simulink model "Copy_of_MPC_control"  (R2018a)
settings: Solver=FixedStepAuto  StartTime=0  StopTime=Tend  FixedStep=0.001  RelTol=5e-3
model workspace (MAT data in the model file):
  A_mu = 10
  B_reff = 8.386
  Cz = 7766.25
  DCT_Param : struct (value not decoded)
  D_reff = 0.25826
  Downshift_Speeds = [9.5625 12.9375 16.3125 19.6875 23.0625 26.4375 29.8125 33.1875 36.5625 39.9375 43.3125 46.6875 ... (28 elements, 4x7)]
  Pedal_Positions = [0.1 0.4 0.5 0.9]
  SUS : struct (value not decoded)
  Upshift_Speeds = [12.9375 16.3125 19.6875 33 26.4375 29.8125 33.1875 52.5 39.9375 43.3125 46.6875 77.25 ... (28 elements, 4x7)]
  VEH : struct (value not decoded)
  V_o = 16.7
  V_xlow = 1
  WH : struct (value not decoded)
  a = 1.4
  alpha_max = 1.5
  alpha_min = -1.5
  b = 1.8
  c_zo = 209651
  epsilon = 0.1
  h = 0.134
  path : struct (value not decoded)
  pio = 220000
  q_Fcx = 0
  q_Fz2 = 15.4
  q_Fzy = 0
  q_reo = 0.9974
  q_sx1 = -0.007764
  q_sx10 = 0.2824
  q_sx11 = 5.349
  q_sx12 = 0
  q_sx13 = 0
  q_sx14 = 0
  q_sx2 = 1.1915
  q_sx3 = 0.013948
  q_sx4 = 4.912
  q_sx5 = 1.02
  q_sx6 = 22.83
  q_sx7 = 0.7104
  q_sx8 = -0.023393
  q_sx9 = 0.6581
  q_sy1 = 0.00702
  q_sy2 = 0
  q_sy3 = 0.001515
  q_sy4 = 8.514e-05
  q_sy5 = 0
  q_sy6 = 0
  q_sy7 = 0.9008
  q_sy8 = -0.4089
  q_v1 = 0.0007742
  q_v2 = 0.04667
  r_Bx1 = 12.531
  r_Bx2 = 9.532
  r_Bx3 = 0
  r_By1 = 10.615
  r_By2 = 7.705
  r_By3 = 3.433e-06
  r_By4 = 0
  r_Cx1 = 1.019
  r_Cy1 = 1.0585
  r_Ex1 = -0.4487
  r_Ex2 = -0.4726
  r_Ey1 = 0.3132
  r_Ey2 = 7.63e-06
  r_Hx1 = 0.0002374
  r_Hy1 = 0.011646
  r_Hy2 = 7.63e-06
  r_Vy1 = 0.05654
  r_Vy2 = 7.63e-06
  r_Vy3 = 0
  r_Vy4 = 99.9
  r_Vy5 = 2
  r_Vy6 = 15.814
  r_o = 0.3135
  vehWidth = 2
  w = 1
symbols that are objects in the model workspace (value not decoded): VEH
undefined symbols (not defined in the file): C_Brake, C_Final, C_Front, C_Front_1, C_Front_2, C_Middle, C_out_Brake, C_out_Final, C_out_Front, C_out_Front_1, C_out_Front_2, C_out_Middle, Co, Cok_Brake, Cok_Final, Cok_Front_1, Cok_Front_2, Cok_Middle, Cso, D_out_Brake, D_out_Final, D_out_Front, D_out_Front_1, D_out_Front_2, D_out_Middle, Earlytochange, Earlytochange2, F, F_Brake, F_Final, F_Front, F_Front_1, F_Front_2, F_Middle, Fs, G_Brake, G_Final, G_Front_1, G_Front_2, G_Middle, G_sys_Brake, G_sys_Final, G_sys_Front, G_sys_Front_1, G_sys_Front_2, G_sys_Middle, Gd, Gd_Brake, Gd_Final, Gd_Front, Gd_Front_1, Gd_Front_2, Gd_Middle, Go, Gsd, Gso, H_Brake, H_Final, H_Front_1, H_Front_2 ... (+60)
libraries: simulink x10, sim3dlib x4, autolibutils x2, vehdynlibviscommon x2
(part 4 of 8)

== system Copy_of_MPC_control/Visualization/3D Engine/3D Engine ==
  VehFdbk : Inport
  3D Body Offset : Constant  Value=single(0.0112)  OutDataTypeStr=single
  Add1 : Sum  Inputs=-+
  Add3 : Sum  Inputs=-+-
  Bus Selector : BusSelector  OutputSignals=Body.X,Body.Y,Body.Z,Body.phi,Body.theta,Body.psi
  Bus Selector2 : BusSelector  OutputSignals=Wheels.zAxle,Wheels.omega,Driveline.WhlAng
  Bus Selector3 : BusSelector  OutputSignals=Body.ZHP
  Constant1 : Constant  Value=zeros(4,1)  OutDataTypeStr=single
  Constant2 : Constant  Value=0  OutDataTypeStr=single
  Constant8 : Constant  Value=h
  Data Type Conversion{1,4..10,12} (9 alike) : DataTypeConversion  OutDataTypeStr=single
  Demux{,1..3} (4 alike) : Demux
  Integrator : Integrator  WrapState=on  WrappedStateUpperValue=2*pi  WrappedStateLowerValue=0  ZeroCross=off
  Part Rotation Concatenation : Subsystem
  Part Translation Concatenation : Subsystem
  Rate Transition : RateTransition  OutPortSampleTime=dt3D
  Scale : Subsystem
  Simulation 3D Engine 1 : sim3dlib/Simulation 3D Config  Priority=1  ProjectFormat=Executable  ProjectName=VehicleSimulation.exe  SceneDesc=Straight road  OpVisEn=off  Ts=dt3D
      settings: AttributesFormatString=Priority: %<Priority>
  Unary Minus : UnaryMinus
  Vehicle Actor Transform Set : sim3dlib/Simulation 3D Actor Transform Set  ActorTag=SimulinkVehicle1  ActorType=Passenger vehicle  PassVehMesh=Muscle car  VehColor=Red  NumberOfParts=5  CustNumOfParts=3  Translation=[0 0 1; 0 0 0; 0 0 0; 0 0 0; 0 0 0]  Rotation=[0 0 0; 0 0 0; 0 0 0; 0 0 0; 0 0 0]  Scale=[1 1 1; 1 1 1; 1 1 1; 1 1 1; 1 1 1]  Ts=dt3D
  wires:
  Unary Minus/1 -> Integrator/1
  Bus Selector3/1 -> Add3/2  "<ZHP>"
  Add3/1 -> Data Type Conversion12/1
  Bus Selector2/1 -> Add3/3  "<zAxle>"
  Constant8/1 -> Add3/1
  Rate Transition/1 -> Bus Selector/1, Bus Selector3/1, Bus Selector2/1
  Scale/1(ScaleOut) -> Vehicle Actor Transform Set/3
  Demux/4 -> Part Rotation Concatenation/7(WheelRearRight Ptich)
  Demux/3 -> Part Rotation Concatenation/6(WheelRearLeft Pitch)
  Demux/2 -> Part Rotation Concatenation/5(WheelFrontRight Pitch)
  Demux/1 -> Part Rotation Concatenation/4(WheelFrontLeft Pitch)
  Constant1/1 -> Demux2/1
  Bus Selector/4 -> Data Type Conversion7/1  "<phi>"
  Data Type Conversion6/1 -> Add1/1
  Part Rotation Concatenation/1(ConcatOut) -> Vehicle Actor Transform Set/2
  Part Translation Concatenation/1(ConcatOut) -> Vehicle Actor Transform Set/1
  Data Type Conversion12/1 -> Demux3/1
  Demux3/4 -> Part Translation Concatenation/15(WheelRearRightZ)
  Demux3/3 -> Part Translation Concatenation/14(WheelRearLeftZ)
  Demux3/1 -> Part Translation Concatenation/12(WheelFrontLeftZ)
  Demux3/2 -> Part Translation Concatenation/13(WheelFrontRightZ)
  VehFdbk/1 -> Rate Transition/1
  Add1/1 -> Part Translation Concatenation/3(BodyZ)
  3D Body Offset/1 -> Add1/2
  Demux1/4 -> Part Rotation Concatenation/15(WheelRearRight Yaw)
  Demux1/3 -> Part Rotation Concatenation/14(WheelRearLeft Yaw)
  Demux2/1 -> Part Rotation Concatenation/8(WheelFrontLeft Roll)
  Demux2/2 -> Part Rotation Concatenation/9(WheelFrontRight Roll)
  Demux2/3 -> Part Rotation Concatenation/10(WheelRearLeft Roll)
  Demux2/4 -> Part Rotation Concatenation/11(WheelRearRight Roll)
  Bus Selector2/3 -> Data Type Conversion9/1  "<WhlAng>"
  Bus Selector2/2 -> Unary Minus/1  "<omega>"
  Data Type Conversion9/1 -> Demux1/1
  Demux1/1 -> Part Rotation Concatenation/12(WheelFrontLeft Yaw)
  Demux1/2 -> Part Rotation Concatenation/13(WheelFrontRight Yaw)
  Integrator/1 -> Data Type Conversion1/1
  Data Type Conversion1/1 -> Demux/1
  Data Type Conversion8/1 -> Part Rotation Concatenation/2(Body Ptich)
  Data Type Conversion5/1 -> Part Translation Concatenation/2(BodyY)
  Data Type Conversion10/1 -> Part Rotation Concatenation/3(Body Yaw)
  Constant2/1 -> Part Translation Concatenation/5(WheelFrontRightX), Part Translation Concatenation/6(WheelRearLeftX), Part Translation Concatenation/7(WheelRearRightX), Part Translation Concatenation/8(WheelFrontLeftY), Part Translation Concatenation/9(WheelFrontRightY), Part Translation Concatenation/10(WheelRearLeftY), Part Translation Concatenation/11(WheelRearRightY), Part Translation Concatenation/4(WheelFrontLeftX)
  Data Type Conversion4/1 -> Part Translation Concatenation/1(BodyX)
  Data Type Conversion7/1 -> Part Rotation Concatenation/1(Body Roll)
  Bus Selector/1 -> Data Type Conversion4/1  "<X>"
  Bus Selector/2 -> Data Type Conversion5/1  "<Y>"
  Bus Selector/3 -> Data Type Conversion6/1  "<Z>"
  Bus Selector/6 -> Data Type Conversion10/1  "<psi>"
  Bus Selector/5 -> Data Type Conversion8/1  "<theta>"

== system Copy_of_MPC_control/Visualization/3D Engine/3D Engine Disabled ==
  VehFdbk : Inport
  Terminator : Terminator
  wires:
  VehFdbk/1 -> Terminator/1

== system Copy_of_MPC_control/all_system/Controllers1/Brake Controller ==
  BrkPrsCmd : Inport
  xdot : Inport  Port=2
  kappa : Inport  Port=3
  Abs : Abs  ZeroCross=off
  Brake Pressure Control : Subsystem  Variant=on  OverrideUsingVariant=0
  Constant1 : Constant  Value=-20
  Gain3 : Gain
  Integrator2 : Integrator  LimitOutput=on  UpperSaturationLimit=1  LowerSaturationLimit=0
  Saturation : Saturate  UpperLimit=1  LowerLimit=0  ZeroCross=off
  Switch1 : Switch  Criteria=u2 > Threshold  Threshold=.1
  Vector Concatenate2 : Concatenate  NumInputs=4
  PCmd : Outport
  wires:
  Constant1/1 -> Switch1/3
  Gain3/1 -> Switch1/1
  Saturation/1 -> Brake Pressure Control/3(<Kappa>)  "Kappa"
  Brake Pressure Control/1(PCmd) -> PCmd/1
  kappa/1 -> Abs/1
  Integrator2/1 -> Vector Concatenate2/4, Vector Concatenate2/3, Vector Concatenate2/2, Vector Concatenate2/1
  xdot/1 -> Brake Pressure Control/2(xdot)
  Abs/1 -> Saturation/1
  Vector Concatenate2/1 -> Brake Pressure Control/1(Pref)  "Reference P"
  BrkPrsCmd/1 -> Switch1/2, Gain3/1
  Switch1/1 -> Integrator2/1

== system Copy_of_MPC_control/all_system/Controllers1/ECU ==
  <Accel> : Inport
  Acc to Torque Request : Gain  Gain=150
  Trq Cmd : Outport
  wires:
  <Accel>/1 -> Acc to Torque Request/1
  Acc to Torque Request/1 -> Trq Cmd/1

== system Copy_of_MPC_control/all_system/Controllers1/Transmission Controller ==
  Acc : Inport
  EngSpd : Inport  Port=2  Unit=rad/s
  PropShaftSpd : Inport  Port=3
  10ms Function-Call Generator : simulink/Ports & Subsystems/Function-Call Generator  sample_time=Fcncal_transctrl_Ts  numberOfIterations=1
  Rate Transition{,1..3} (4 alike) : RateTransition
  Signal Specification : SignalSpecification  Unit=rpm
  TCM : Subsystem
  Unit Conversion : UnitConversion
  Gear : Outport
  wires:
  TCM/1(Gear Select) -> Rate Transition3/1
  Rate Transition/1 -> TCM/1(AccCmd)
  10ms Function-Call Generator/1 -> TCM/Trigger
  Acc/1 -> Rate Transition/1
  PropShaftSpd/1 -> Rate Transition2/1
  Rate Transition1/1 -> TCM/2(EngSpd)
  Rate Transition2/1 -> TCM/3(VehSpdFdbk)
  Rate Transition3/1 -> Gear/1
  Unit Conversion/1 -> Signal Specification/1
  Signal Specification/1 -> Rate Transition1/1  "EngSpd"
  EngSpd/1 -> Unit Conversion/1

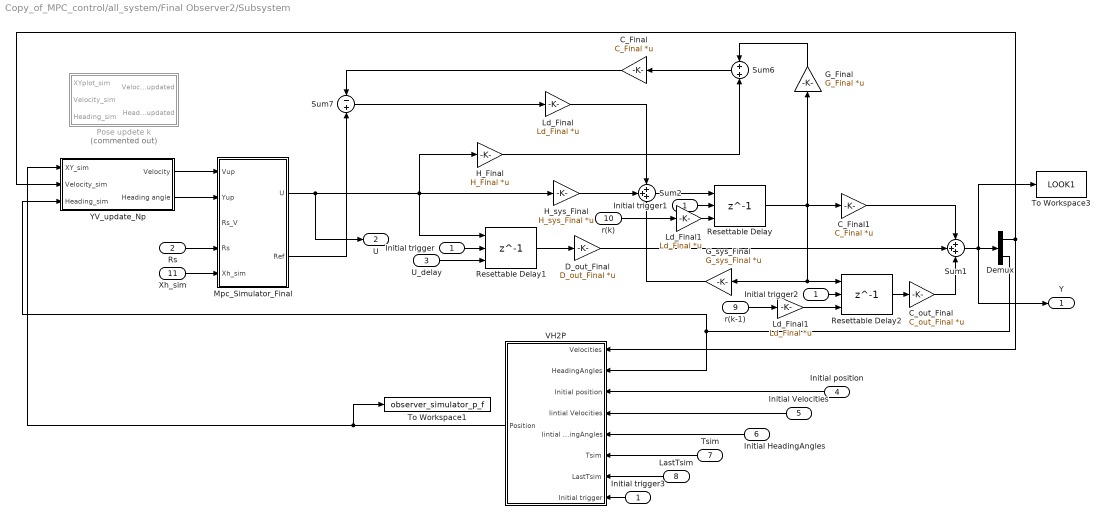
== system Copy_of_MPC_control/all_system/Final Observer2/Subsystem ==
  Initial trigger : Inport
  Rs : Inport  Port=2
  U_delay : Inport  Port=3
  Initial position : Inport  Port=4
  Initial Velocities : Inport  Port=5
  Initial HeadingAngles : Inport  Port=6
  Tsim : Inport  Port=7
  LastTsim : Inport  Port=8
  r(k-1) : Inport  Port=9
  r(k) : Inport  Port=10
  Xh_sim : Inport  Port=11
  C_Final : Gain  Gain=C_Final  Multiplication=Matrix(K*u) (u vector)
  C_Final1 : Gain  Gain=C_Final  Multiplication=Matrix(K*u) (u vector)
  C_out_Final : Gain  Gain=C_out_Final  Multiplication=Matrix(K*u) (u vector)
  D_out_Final : Gain  Gain=D_out_Final  Multiplication=Matrix(K*u) (u vector)
  Demux : Demux  Outputs=2
  G_Final : Gain  Gain=G_Final  Multiplication=Matrix(K*u) (u vector)
  G_sys_Final : Gain  Gain=G_sys_Final  Multiplication=Matrix(K*u) (u vector)
  H_Final : Gain  Gain=H_Final  Multiplication=Matrix(K*u) (u vector)
  H_sys_Final : Gain  Gain=H_sys_Final  Multiplication=Matrix(K*u) (u vector)
  Initial trigger1 : InportShadow
  Initial trigger2 : InportShadow
  Initial trigger3 : InportShadow
  Ld_Final : Gain  Gain=Ld_Final  Multiplication=Matrix(K*u) (u vector)
  Ld_Final1 : Gain  Gain=Ld_Final  Multiplication=Matrix(K*u) (u vector)
  "Ld_Final1 " : Gain  Gain=Ld_Final  Multiplication=Matrix(K*u) (u vector)
  Mpc_Simulator_Final : Subsystem
  Pose updete k : Subsystem  Commented=on
  Resettable Delay : Delay  DelayLength=1  InitialConditionSource=Input port  ExternalReset=Falling  SampleTime=Ts
      settings: InputPortMap=u0,r5,p4
  Resettable Delay1 : Delay  DelayLength=1  InitialConditionSource=Input port  ExternalReset=Falling  SampleTime=Ts
      settings: InputPortMap=u0,r5,p4
  Resettable Delay2 : Delay  DelayLength=1  InitialConditionSource=Input port  ExternalReset=Falling  SampleTime=Ts
      settings: InputPortMap=u0,r5,p4
  Sum1 : Sum  Inputs=+++
  Sum2 : Sum  Inputs=+++
  Sum6 : Sum
  Sum7 : Sum  Inputs=-+
  To Workspace1 : ToWorkspace  VariableName=observer_simulator_p_f  SampleTime=Ts
  To Workspace3 : ToWorkspace  VariableName=LOOK1  SampleTime=Ts
  VH2P : Subsystem
  YV_update_Np : Subsystem  TreatAsAtomicUnit=on
  Y : Outport
  U : Outport  Port=2
  wires:
  U_delay/1 -> Resettable Delay1/3
  Initial position/1 -> VH2P/3(Initial position)
  Mpc_Simulator_Final/1(U) -> U/1, Resettable Delay1/1, H_sys_Final/1, H_Final/1
  Resettable Delay/1 -> G_sys_Final/1, Resettable Delay2/1, C_Final1/1, G_Final/1
  Sum7/1 -> Ld_Final/1
  C_Final1/1 -> Sum1/1
  Rs/1 -> Mpc_Simulator_Final/4(Rs)
  Demux/1 -> YV_update_Np/2(Velocity_sim), VH2P/1(Velocities)
  Demux/2 -> YV_update_Np/3(Heading_sim), VH2P/2(HeadingAngles)
  Resettable Delay1/1 -> D_out_Final/1
  LastTsim/1 -> VH2P/7(LastTsim)
  Ld_Final/1 -> Sum2/1
  Initial Velocities/1 -> VH2P/4(Iintial Velocities)
  D_out_Final/1 -> Sum1/2
  YV_update_Np/1(Velocity) -> Mpc_Simulator_Final/1(Vup)
  r(k)/1 -> "Ld_Final1 "/1
  Resettable Delay2/1 -> C_out_Final/1
  G_sys_Final/1 -> Sum2/3
  r(k-1)/1 -> Ld_Final1/1
  C_Final/1 -> Sum7/1
  Sum2/1 -> Resettable Delay/1
  VH2P/1(Position) -> YV_update_Np/1(XY_sim), To Workspace1/1
  YV_update_Np/2(Heading angle) -> Mpc_Simulator_Final/2(Yup)
  Xh_sim/1 -> Mpc_Simulator_Final/5(Xh_sim)
  Tsim/1 -> VH2P/6(Tsim)
  "Ld_Final1 "/1 -> Resettable Delay/3
  Initial HeadingAngles/1 -> VH2P/5(Iintial HeadingAngles)
  G_Final/1 -> Sum6/1
  H_Final/1 -> Sum6/2
  C_out_Final/1 -> Sum1/3
  Sum1/1 -> Y/1, To Workspace3/1, Demux/1
  Sum6/1 -> C_Final/1
  Mpc_Simulator_Final/2(Ref) -> Sum7/2
  H_sys_Final/1 -> Sum2/2
  Ld_Final1/1 -> Resettable Delay2/3
  Initial trigger/1 -> Resettable Delay1/2
  Initial trigger1/1 -> Resettable Delay/2
  Initial trigger2/1 -> Resettable Delay2/2
  Initial trigger3/1 -> VH2P/8(Initial trigger)

== system Copy_of_MPC_control/all_system/Final_simulator1/Mpc_Simulator_Final ==
  Vup : Inport  SampleTime=Ts  LockScale=on
  Yup : Inport  Port=2  SampleTime=Ts  LockScale=on
  Rs_V : Inport  Port=3  SampleTime=Ts  LockScale=on
  Rs : Inport  Port=4  SampleTime=Ts  LockScale=on
  Xh_sim : Inport  Port=5
  Clock : Clock
  Constant1 : Constant  Value=M  VectorParams1D=off  SampleTime=-1
  Constant2 : Constant  Value=Np  SampleTime=-1
  Constant3 : Constant  Value=Upd_end  VectorParams1D=off  SampleTime=-1
  Constant4 : Constant  Value=Qc  VectorParams1D=off  SampleTime=-1
  Constant5 : Constant  Value=phi_Final  VectorParams1D=off  SampleTime=-1
  Constant6 : Constant  Value=JE_Final  VectorParams1D=off  SampleTime=-1
  F_Final : Gain  Gain=F_Final  Multiplication=Matrix(K*u) (u vector)
  MATLAB Function : MATLAB Function  TreatAsAtomicUnit=on  SystemSampleTime=Ts
  Unit Delay : UnitDelay  InitialCondition=[0;0]  SampleTime=Ts
  U : Outport
  Ref : Outport  Port=2
  lambda : Outport  Port=3
  wires:
  Unit Delay/1 -> MATLAB Function/13(u)
  MATLAB Function/2(U) -> U/1, Unit Delay/1
  MATLAB Function/1(Ref) -> Ref/1
  Xh_sim/1 -> F_Final/1
  Constant4/1 -> MATLAB Function/5(Qc)
  Constant5/1 -> MATLAB Function/4(phi)
  Constant6/1 -> MATLAB Function/1(JE)
  Constant2/1 -> MATLAB Function/3(Np)
  Rs_V/1 -> MATLAB Function/10(Rs_V)
  Yup/1 -> MATLAB Function/7(Yup)
  Constant1/1 -> MATLAB Function/2(M)
  Clock/1 -> MATLAB Function/11(Tsim)
  F_Final/1 -> MATLAB Function/6(Fxh)
  Vup/1 -> MATLAB Function/8(Vup)
  Rs/1 -> MATLAB Function/9(Rs)
  Constant3/1 -> MATLAB Function/12(Upd_end)
  MATLAB Function/3(lambda) -> lambda/1

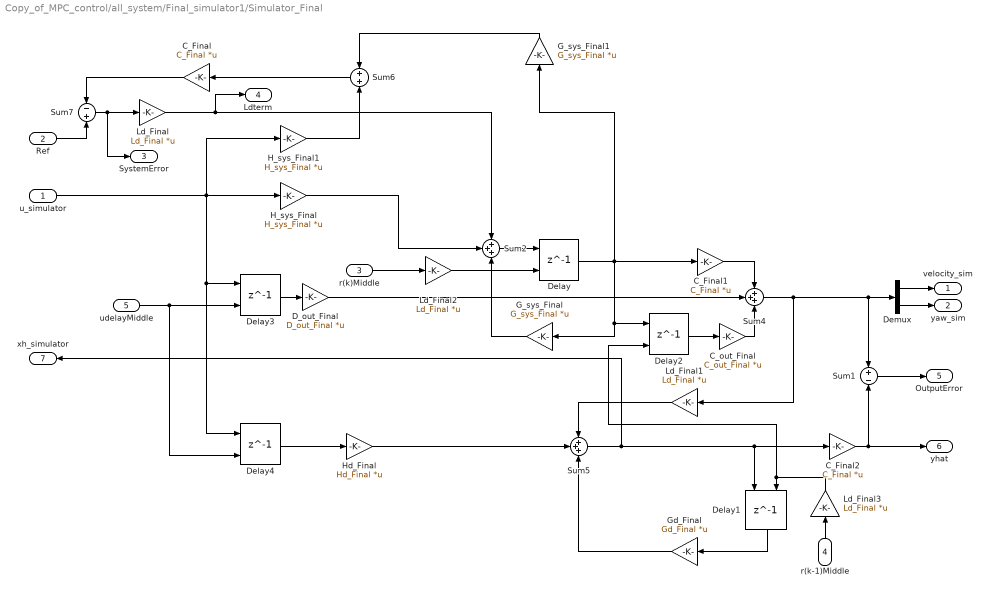
== system Copy_of_MPC_control/all_system/Final_simulator1/Simulator_Final ==
  u_simulator : Inport
  Ref : Inport  Port=2
  r(k)Middle : Inport  Port=3
  r(k-1)Middle : Inport  Port=4
  udelayMiddle : Inport  Port=5
  C_Final : Gain  Gain=C_Final  Multiplication=Matrix(K*u) (u vector)
  C_Final1 : Gain  Gain=C_Final  Multiplication=Matrix(K*u) (u vector)
  C_Final2 : Gain  Gain=C_Final  Multiplication=Matrix(K*u) (u vector)
  C_out_Final : Gain  Gain=C_out_Final  Multiplication=Matrix(K*u) (u vector)
  D_out_Final : Gain  Gain=D_out_Final  Multiplication=Matrix(K*u) (u vector)
  Delay{,1..4} (5 alike) : Delay  DelayLength=1  InitialConditionSource=Input port  InitialCondition=0  SampleTime=Ts
      settings: InputPortMap=u0,p4
  Demux : Demux  Outputs=2
  G_sys_Final : Gain  Gain=G_sys_Final  Multiplication=Matrix(K*u) (u vector)
  G_sys_Final1 : Gain  Gain=G_sys_Final  Multiplication=Matrix(K*u) (u vector)
  Gd_Final : Gain  Gain=Gd_Final  Multiplication=Matrix(K*u) (u vector)
  H_sys_Final : Gain  Gain=H_sys_Final  Multiplication=Matrix(K*u) (u vector)
  H_sys_Final1 : Gain  Gain=H_sys_Final  Multiplication=Matrix(K*u) (u vector)
  Hd_Final : Gain  Gain=Hd_Final  Multiplication=Matrix(K*u) (u vector)
  Ld_Final{,1..3} (4 alike) : Gain  Gain=Ld_Final  Multiplication=Matrix(K*u) (u vector)
  Sum1 : Sum  Inputs=+-
  Sum2 : Sum  Inputs=+++
  Sum4 : Sum  Inputs=+++
  Sum5 : Sum  Inputs=+++
  Sum6 : Sum
  Sum7 : Sum  Inputs=-+
  velocity_sim : Outport
  yaw_sim : Outport  Port=2
  SystemError : Outport  Port=3
  Ldterm : Outport  Port=4
  OutputError : Outport  Port=5
  yhat : Outport  Port=6
  xh_simulator : Outport  Port=7
  wires:
  H_sys_Final/1 -> Sum2/2
  D_out_Final/1 -> Sum4/2
  Delay1/1 -> Gd_Final/1
  u_simulator/1 -> Delay4/1, Delay3/1, H_sys_Final1/1, H_sys_Final/1
  Ld_Final/1 -> Ldterm/1, Sum2/1
  G_sys_Final1/1 -> Sum6/1
  Sum2/1 -> Delay/1
  C_Final/1 -> Sum7/1
  H_sys_Final1/1 -> Sum6/2
  Delay3/1 -> D_out_Final/1
  Ref/1 -> Sum7/2
  Delay4/1 -> Hd_Final/1
  Delay2/1 -> C_out_Final/1
  Ld_Final1/1 -> Sum5/1
  Delay/1 -> Delay2/1, G_sys_Final/1, G_sys_Final1/1, C_Final1/1
  Hd_Final/1 -> Sum5/2
  C_out_Final/1 -> Sum4/3
  Sum5/1 -> xh_simulator/1, C_Final2/1, Delay1/1
  Sum7/1 -> SystemError/1, Ld_Final/1
  C_Final1/1 -> Sum4/1
  G_sys_Final/1 -> Sum2/3
  Sum6/1 -> C_Final/1
  Gd_Final/1 -> Sum5/3
  Demux/2 -> yaw_sim/1
  Demux/1 -> velocity_sim/1
  Sum4/1 -> Sum1/1, Demux/1, Ld_Final1/1
  C_Final2/1 -> yhat/1, Sum1/2
  Sum1/1 -> OutputError/1
  Ld_Final2/1 -> Delay/2
  r(k)Middle/1 -> Ld_Final2/1
  r(k-1)Middle/1 -> Ld_Final3/1
  Ld_Final3/1 -> Delay2/2, Delay1/2
  udelayMiddle/1 -> Delay4/2, Delay3/2

== system Copy_of_MPC_control/all_system/Final_simulator1/VH2P ==
  Velocities : Inport
  HeadingAngles : Inport  Port=2
  PositionfromMiddle : Inport  Port=3
  VelocitiesfromMiddle : Inport  Port=4
  HeadingAnglesfromMiddle : Inport  Port=5
  T_sim : Inport  Port=6
  LastT_sim : Inport  Port=7
  Resettable Delay : Delay  DelayLength=1  InitialConditionSource=Input port  ExternalReset=Rising  SampleTime=Ts
      settings: InputPortMap=u0,r5,p4
  Resettable Delay1 : Delay  DelayLength=1  InitialConditionSource=Input port  ExternalReset=Rising  SampleTime=Ts
      settings: InputPortMap=u0,r5,p4
  Resettable Delay2 : Delay  DelayLength=1  InitialConditionSource=Input port  ExternalReset=Rising  SampleTime=Ts
      settings: InputPortMap=u0,r5,p4
  Trigger : Subsystem
  YV2P : MATLAB Function  TreatAsAtomicUnit=on  SystemSampleTime=Ts
  Position : Outport
  wires:
  YV2P/1(Position) -> Resettable Delay/1, Position/1
  LastT_sim/1 -> YV2P/6(LastTsim)
  Velocities/1 -> YV2P/1(Velocity), Resettable Delay1/1
  Resettable Delay1/1 -> YV2P/3(LastVelocity)
  HeadingAngles/1 -> YV2P/2(Yaw), Resettable Delay2/1
  Resettable Delay2/1 -> YV2P/4(LastYaw)
  Resettable Delay/1 -> YV2P/7(Lastpostion)
  Trigger/1(Trig) -> Resettable Delay2/2, Resettable Delay1/2, Resettable Delay/2
  PositionfromMiddle/1 -> Resettable Delay/3
  HeadingAnglesfromMiddle/1 -> Resettable Delay2/3
  VelocitiesfromMiddle/1 -> Resettable Delay1/3
  T_sim/1 -> YV2P/5(Tsim)

== system Copy_of_MPC_control/all_system/Final_simulator1/YV_update_Np ==
  XY_sim : Inport
  Velocity_sim : Inport  Port=2
  Heading_sim : Inport  Port=3
  From Workspace1 : FromWorkspace  VariableName=T_sim  SampleTime=Ts
  From Workspace3 : FromWorkspace  VariableName=XY_Ref_Upd  SampleTime=Ts
  MATLAB Function2 : MATLAB Function  TreatAsAtomicUnit=on  SystemSampleTime=Ts
  Unit Delay1 : UnitDelay  SampleTime=Ts
  Unit Delay4 : UnitDelay  SampleTime=Ts
  Unit Delay5 : UnitDelay  SampleTime=Ts
  Velocity : Outport
  Heading angle : Outport  Port=2
  wires:
  MATLAB Function2/1(Velocity_updated) -> Velocity/1
  From Workspace3/1 -> MATLAB Function2/1(XY_ref)
  MATLAB Function2/2(Heading_updated) -> Heading angle/1
  From Workspace1/1 -> MATLAB Function2/8(Tsim)
  XY_sim/1 -> Unit Delay1/1, MATLAB Function2/2(XY_sim)
  Velocity_sim/1 -> MATLAB Function2/4(Velocity_sim), Unit Delay5/1
  Heading_sim/1 -> MATLAB Function2/6(Yaw_sim), Unit Delay4/1
  Unit Delay1/1 -> MATLAB Function2/3(LastXY_sim)
  Unit Delay5/1 -> MATLAB Function2/5(LastVelocity_sim)
  Unit Delay4/1 -> MATLAB Function2/7(LastYaw_sim)

== system Copy_of_MPC_control/all_system/Front_simulator1/Mpc_Simulator_Front ==
  Vup : Inport  SampleTime=Ts  LockScale=on
  Yup : Inport  Port=2  SampleTime=Ts  LockScale=on
  Rs_V : Inport  Port=3  SampleTime=Ts  LockScale=on
  Xh_sim : Inport  Port=4
  Rs : Inport  Port=5  SampleTime=Ts  LockScale=on
  Clock : Clock
  Constant1 : Constant  Value=M  VectorParams1D=off  SampleTime=-1
  Constant2 : Constant  Value=Np  SampleTime=-1
  Constant4 : Constant  Value=Qc  VectorParams1D=off  SampleTime=-1
  Constant5 : Constant  Value=phi_Front  VectorParams1D=off  SampleTime=-1
  Constant6 : Constant  Value=JE_Front  VectorParams1D=off  SampleTime=-1
  F_Front : Gain  Gain=F_Front  Multiplication=Matrix(K*u) (u vector)
  MATLAB Function : MATLAB Function  TreatAsAtomicUnit=on  SystemSampleTime=Ts
  Unit Delay : UnitDelay  InitialCondition=[0;0]  SampleTime=Ts
  U : Outport
  Ref : Outport  Port=2
  lambda : Outport  Port=3
  wires:
  Unit Delay/1 -> MATLAB Function/12(u)
  MATLAB Function/2(U) -> U/1, Unit Delay/1
  MATLAB Function/1(Ref) -> Ref/1
  Xh_sim/1 -> F_Front/1
  Constant4/1 -> MATLAB Function/5(Qc)
  Constant5/1 -> MATLAB Function/4(phi)
  Constant6/1 -> MATLAB Function/1(JE)
  Constant2/1 -> MATLAB Function/3(Np)
  Rs_V/1 -> MATLAB Function/10(Rs_V)
  Yup/1 -> MATLAB Function/7(Yup)
  Constant1/1 -> MATLAB Function/2(M)
  Clock/1 -> MATLAB Function/11(Tsim)
  F_Front/1 -> MATLAB Function/6(Fxh)
  Vup/1 -> MATLAB Function/8(Vup)
  Rs/1 -> MATLAB Function/9(Rs)
  MATLAB Function/3(lambda) -> lambda/1

== system Copy_of_MPC_control/all_system/Front_simulator1/Simulator_Front ==
  u_simulator : Inport
  Ref : Inport  Port=2
  C_Front : Gain  Gain=C_Front  Multiplication=Matrix(K*u) (u vector)
  C_Front1 : Gain  Gain=C_Front  Multiplication=Matrix(K*u) (u vector)
  C_Front2 : Gain  Gain=C_Front  Multiplication=Matrix(K*u) (u vector)
  C_out_Front : Gain  Gain=C_out_Front  Multiplication=Matrix(K*u) (u vector)
  D_out_Front : Gain  Gain=D_out_Front  Multiplication=Matrix(K*u) (u vector)
  Demux : Demux  Outputs=2
  G_sys_Front : Gain  Gain=G_sys_Front  Multiplication=Matrix(K*u) (u vector)
  G_sys_Front1 : Gain  Gain=G_sys_Front  Multiplication=Matrix(K*u) (u vector)
  Gd_Front : Gain  Gain=Gd_Front  Multiplication=Matrix(K*u) (u vector)
  H_sys_Front : Gain  Gain=H_sys_Front  Multiplication=Matrix(K*u) (u vector)
  H_sys_Front1 : Gain  Gain=H_sys_Front  Multiplication=Matrix(K*u) (u vector)
  Hd_Front : Gain  Gain=Hd_Front  Multiplication=Matrix(K*u) (u vector)
  Ld_Front : Gain  Gain=Ld_Front  Multiplication=Matrix(K*u) (u vector)
  Ld_Front1 : Gain  Gain=Ld_Front  Multiplication=Matrix(K*u) (u vector)
  Sum1 : Sum  Inputs=+-
  Sum2 : Sum  Inputs=+++
  Sum4 : Sum  Inputs=+++
  Sum5 : Sum  Inputs=+++
  Sum6 : Sum
  Sum7 : Sum  Inputs=-+
  Unit Delay{2,4..6,9} (5 alike) : UnitDelay  SampleTime=Ts
  velocity_sim : Outport
  yaw_sim : Outport  Port=2
  xh_simulator : Outport  Port=3
  SystemError : Outport  Port=4
  Ldterm : Outport  Port=5
  OutputError : Outport  Port=6
  yhat : Outport  Port=7
  wires:
  H_sys_Front/1 -> Sum2/2
  D_out_Front/1 -> Sum4/2
  Unit Delay5/1 -> Gd_Front/1
  u_simulator/1 -> Unit Delay9/1, Unit Delay4/1, H_sys_Front1/1, H_sys_Front/1
  Ld_Front/1 -> Ldterm/1, Sum2/1
  G_sys_Front1/1 -> Sum6/1
  Sum2/1 -> Unit Delay2/1
  C_Front/1 -> Sum7/1
  H_sys_Front1/1 -> Sum6/2
  Unit Delay4/1 -> D_out_Front/1
  Ref/1 -> Sum7/2
  Unit Delay9/1 -> Hd_Front/1
  Unit Delay6/1 -> C_out_Front/1
  Ld_Front1/1 -> Sum5/1
  Unit Delay2/1 -> Unit Delay6/1, G_sys_Front/1, C_Front1/1, G_sys_Front1/1
  Hd_Front/1 -> Sum5/2
  C_out_Front/1 -> Sum4/3
  Sum5/1 -> xh_simulator/1, C_Front2/1, Unit Delay5/1
  Sum7/1 -> SystemError/1, Ld_Front/1
  C_Front1/1 -> Sum4/1
  G_sys_Front/1 -> Sum2/3
  Sum6/1 -> C_Front/1
  Gd_Front/1 -> Sum5/3
  Demux/2 -> yaw_sim/1
  Demux/1 -> velocity_sim/1
  Sum4/1 -> Sum1/1, Demux/1, Ld_Front1/1
  C_Front2/1 -> yhat/1, Sum1/2
  Sum1/1 -> OutputError/1

== system Copy_of_MPC_control/all_system/Front_simulator1/VH2P ==
  Velocities : Inport
  HeadingAngles : Inport  Port=2
  From Workspace2 : FromWorkspace  VariableName=T_sim  SampleTime=Ts
  Unit Delay4 : UnitDelay  SampleTime=Ts
  Unit Delay5 : UnitDelay  SampleTime=Ts
  Unit Delay6 : UnitDelay  SampleTime=Ts
  Unit Delay7 : UnitDelay  InitialCondition=XYplot(1,:)'  SampleTime=Ts
  YV2P : MATLAB Function  TreatAsAtomicUnit=on  SystemSampleTime=Ts
  Position : Outport
  wires:
  YV2P/1(Position) -> Position/1, Unit Delay7/1
  Unit Delay6/1 -> YV2P/6(LastTsim)
  Velocities/1 -> Unit Delay5/1, YV2P/1(Velocity)
  Unit Delay5/1 -> YV2P/3(LastVelocity)
  HeadingAngles/1 -> YV2P/2(Yaw), Unit Delay4/1
  Unit Delay4/1 -> YV2P/4(LastYaw)
  From Workspace2/1 -> Unit Delay6/1, YV2P/5(Tsim)
  Unit Delay7/1 -> YV2P/7(Lastpostion)

== system Copy_of_MPC_control/all_system/Front_simulator1/YV_update_Np ==
  XY_sim : Inport
  Velocity_sim : Inport  Port=2
  Heading_sim : Inport  Port=3
  From Workspace1 : FromWorkspace  VariableName=T_sim  SampleTime=Ts
  From Workspace3 : FromWorkspace  VariableName=XY_Ref_Upd  SampleTime=Ts
  MATLAB Function2 : MATLAB Function  TreatAsAtomicUnit=on  SystemSampleTime=Ts
  Unit Delay1 : UnitDelay  SampleTime=Ts
  Unit Delay4 : UnitDelay  SampleTime=Ts
  Unit Delay5 : UnitDelay  SampleTime=Ts
  Velocity : Outport
  Heading angle : Outport  Port=2
  wires:
  MATLAB Function2/1(Velocity_updated) -> Velocity/1
  From Workspace3/1 -> MATLAB Function2/1(XY_ref)
  MATLAB Function2/2(Heading_updated) -> Heading angle/1
  From Workspace1/1 -> MATLAB Function2/8(Tsim)
  XY_sim/1 -> Unit Delay1/1, MATLAB Function2/2(XY_sim)
  Velocity_sim/1 -> MATLAB Function2/4(Velocity_sim), Unit Delay5/1
  Heading_sim/1 -> MATLAB Function2/6(Yaw_sim), Unit Delay4/1
  Unit Delay1/1 -> MATLAB Function2/3(LastXY_sim)
  Unit Delay5/1 -> MATLAB Function2/5(LastVelocity_sim)
  Unit Delay4/1 -> MATLAB Function2/7(LastYaw_sim)

== system Copy_of_MPC_control/all_system/Middle Observer2/Observer_state2 ==
  Clock9 : Clock
  Observer_state2 : MATLAB Function  TreatAsAtomicUnit=on  SystemSampleTime=Ts
  Timetochange : Constant  Value=Timetochange  VectorParams1D=off  SampleTime=-1
  Timetochange1 : Constant  Value=Earlytochange  VectorParams1D=off  SampleTime=-1
  state : Outport
  wires:
  Timetochange/1 -> Observer_state2/2(Timetochange)
  Clock9/1 -> Observer_state2/1(timing)
  Observer_state2/1(state) -> state/1
  Timetochange1/1 -> Observer_state2/3(Earlytochange)

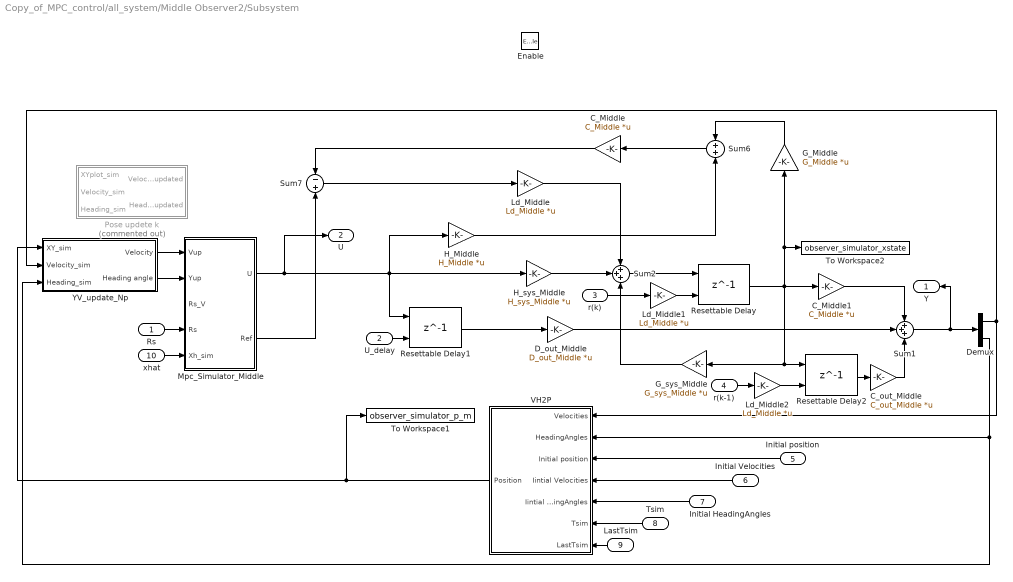
== system Copy_of_MPC_control/all_system/Middle Observer2/Subsystem ==
  Rs : Inport
  U_delay : Inport  Port=2
  r(k) : Inport  Port=3
  r(k-1) : Inport  Port=4
  Initial position : Inport  Port=5
  Initial Velocities : Inport  Port=6
  Initial HeadingAngles : Inport  Port=7
  Tsim : Inport  Port=8
  LastTsim : Inport  Port=9
  xhat : Inport  Port=10
  Enable : EnablePort
  C_Middle : Gain  Gain=C_Middle  Multiplication=Matrix(K*u) (u vector)
  C_Middle1 : Gain  Gain=C_Middle  Multiplication=Matrix(K*u) (u vector)
  C_out_Middle : Gain  Gain=C_out_Middle  Multiplication=Matrix(K*u) (u vector)
  D_out_Middle : Gain  Gain=D_out_Middle  Multiplication=Matrix(K*u) (u vector)
  Demux : Demux  Outputs=2
  G_Middle : Gain  Gain=G_Middle  Multiplication=Matrix(K*u) (u vector)
  G_sys_Middle : Gain  Gain=G_sys_Middle  Multiplication=Matrix(K*u) (u vector)
  H_Middle : Gain  Gain=H_Middle  Multiplication=Matrix(K*u) (u vector)
  H_sys_Middle : Gain  Gain=H_sys_Middle  Multiplication=Matrix(K*u) (u vector)
  Ld_Middle : Gain  Gain=Ld_Middle  Multiplication=Matrix(K*u) (u vector)
  Ld_Middle1 : Gain  Gain=Ld_Middle  Multiplication=Matrix(K*u) (u vector)
  Ld_Middle2 : Gain  Gain=Ld_Middle  Multiplication=Matrix(K*u) (u vector)
  Mpc_Simulator_Middle : Subsystem
  Pose updete k : Subsystem  Commented=on
  Resettable Delay : Delay  DelayLength=1  InitialConditionSource=Input port  SampleTime=Ts
      settings: InputPortMap=u0,p4
  Resettable Delay1 : Delay  DelayLength=1  InitialConditionSource=Input port  SampleTime=Ts
      settings: InputPortMap=u0,p4
  Resettable Delay2 : Delay  DelayLength=1  InitialConditionSource=Input port  SampleTime=Ts
      settings: InputPortMap=u0,p4
  Sum1 : Sum  Inputs=+++
  Sum2 : Sum  Inputs=+++
  Sum6 : Sum
  Sum7 : Sum  Inputs=-+
  To Workspace1 : ToWorkspace  VariableName=observer_simulator_p_m  SampleTime=Ts
  To Workspace2 : ToWorkspace  VariableName=observer_simulator_xstate  SampleTime=Ts
  VH2P : Subsystem
  YV_update_Np : Subsystem  TreatAsAtomicUnit=on
  Y : Outport
  U : Outport  Port=2
  wires:
  Initial position/1 -> VH2P/3(Initial position)
  Sum2/1 -> Resettable Delay/1
  Demux/2 -> YV_update_Np/3(Heading_sim), VH2P/2(HeadingAngles)
  Ld_Middle/1 -> Sum2/1
  Sum7/1 -> Ld_Middle/1
  Mpc_Simulator_Middle/2(Ref) -> Sum7/2
  Rs/1 -> Mpc_Simulator_Middle/4(Rs)
  C_out_Middle/1 -> Sum1/3
  G_Middle/1 -> Sum6/1
  C_Middle/1 -> Sum7/1
  Mpc_Simulator_Middle/1(U) -> U/1, Resettable Delay1/1, H_sys_Middle/1, H_Middle/1
  H_sys_Middle/1 -> Sum2/2
  G_sys_Middle/1 -> Sum2/3
  Resettable Delay2/1 -> C_out_Middle/1
  VH2P/1(Position) -> YV_update_Np/1(XY_sim), To Workspace1/1
  Demux/1 -> YV_update_Np/2(Velocity_sim), VH2P/1(Velocities)
  Resettable Delay/1 -> To Workspace2/1, G_Middle/1, G_sys_Middle/1, Resettable Delay2/1, C_Middle1/1
  H_Middle/1 -> Sum6/2
  Sum1/1 -> Y/1, Demux/1
  Sum6/1 -> C_Middle/1
  D_out_Middle/1 -> Sum1/2
  Resettable Delay1/1 -> D_out_Middle/1
  C_Middle1/1 -> Sum1/1
  YV_update_Np/2(Heading angle) -> Mpc_Simulator_Middle/2(Yup)
  xhat/1 -> Mpc_Simulator_Middle/5(Xh_sim)
  YV_update_Np/1(Velocity) -> Mpc_Simulator_Middle/1(Vup)
  r(k)/1 -> Ld_Middle1/1
  Ld_Middle1/1 -> Resettable Delay/2
  U_delay/1 -> Resettable Delay1/2
  r(k-1)/1 -> Ld_Middle2/1
  Ld_Middle2/1 -> Resettable Delay2/2
  Initial Velocities/1 -> VH2P/4(Iintial Velocities)
  Initial HeadingAngles/1 -> VH2P/5(Iintial HeadingAngles)
  LastTsim/1 -> VH2P/7(LastTsim)
  Tsim/1 -> VH2P/6(Tsim)

== system Copy_of_MPC_control/all_system/Middle_simulator1/Mpc_Simulator_Middle ==
  Vup : Inport  SampleTime=Ts  LockScale=on
  Yup : Inport  Port=2  SampleTime=Ts  LockScale=on
  Rs_V : Inport  Port=3  SampleTime=Ts  LockScale=on
  Rs : Inport  Port=4  SampleTime=Ts  LockScale=on
  Xh_sim : Inport  Port=5
  Clock : Clock
  Constant1 : Constant  Value=M  VectorParams1D=off  SampleTime=-1
  Constant2 : Constant  Value=Np  SampleTime=-1
  Constant3 : Constant  Value=Upd_end  VectorParams1D=off  SampleTime=-1
  Constant4 : Constant  Value=Qc  VectorParams1D=off  SampleTime=-1
  Constant5 : Constant  Value=phi_Middle  VectorParams1D=off  SampleTime=-1
  Constant6 : Constant  Value=JE_Middle  VectorParams1D=off  SampleTime=-1
  F_Middle : Gain  Gain=F_Middle  Multiplication=Matrix(K*u) (u vector)
  MATLAB Function : MATLAB Function  TreatAsAtomicUnit=on  SystemSampleTime=Ts
  Unit Delay : UnitDelay  InitialCondition=[0;0]  SampleTime=Ts
  U : Outport
  Ref : Outport  Port=2
  lambda : Outport  Port=3
  wires:
  Unit Delay/1 -> MATLAB Function/13(u)
  MATLAB Function/2(U) -> U/1, Unit Delay/1
  MATLAB Function/1(Ref) -> Ref/1
  Xh_sim/1 -> F_Middle/1
  Constant4/1 -> MATLAB Function/5(Qc)
  Constant5/1 -> MATLAB Function/4(phi)
  Constant6/1 -> MATLAB Function/1(JE)
  Constant2/1 -> MATLAB Function/3(Np)
  Rs_V/1 -> MATLAB Function/10(Rs_V)
  Yup/1 -> MATLAB Function/7(Yup)
  Constant1/1 -> MATLAB Function/2(M)
  Clock/1 -> MATLAB Function/11(Tsim)
  F_Middle/1 -> MATLAB Function/6(Fxh)
  Vup/1 -> MATLAB Function/8(Vup)
  Rs/1 -> MATLAB Function/9(Rs)
  Constant3/1 -> MATLAB Function/12(Upd_end)
  MATLAB Function/3(lambda) -> lambda/1

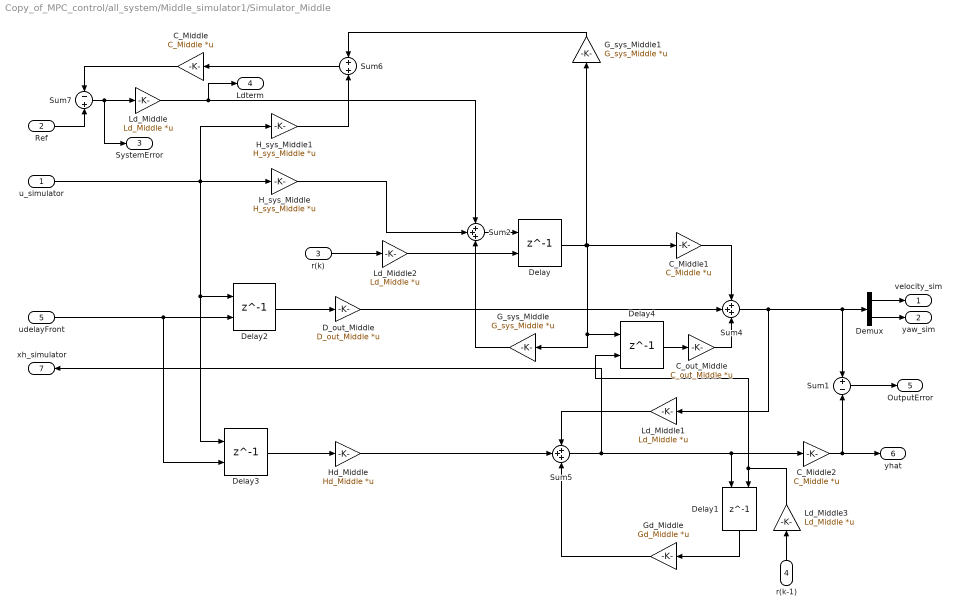
== system Copy_of_MPC_control/all_system/Middle_simulator1/Simulator_Middle ==
  u_simulator : Inport
  Ref : Inport  Port=2
  r(k) : Inport  Port=3
  r(k-1) : Inport  Port=4
  udelayFront : Inport  Port=5
  C_Middle : Gain  Gain=C_Middle  Multiplication=Matrix(K*u) (u vector)
  C_Middle1 : Gain  Gain=C_Middle  Multiplication=Matrix(K*u) (u vector)
  C_Middle2 : Gain  Gain=C_Middle  Multiplication=Matrix(K*u) (u vector)
  C_out_Middle : Gain  Gain=C_out_Middle  Multiplication=Matrix(K*u) (u vector)
  D_out_Middle : Gain  Gain=D_out_Middle  Multiplication=Matrix(K*u) (u vector)
  Delay{,1..4} (5 alike) : Delay  DelayLength=1  InitialConditionSource=Input port  InitialCondition=0  SampleTime=Ts
      settings: InputPortMap=u0,p4
  Demux : Demux  Outputs=2
  G_sys_Middle : Gain  Gain=G_sys_Middle  Multiplication=Matrix(K*u) (u vector)
  G_sys_Middle1 : Gain  Gain=G_sys_Middle  Multiplication=Matrix(K*u) (u vector)
  Gd_Middle : Gain  Gain=Gd_Middle  Multiplication=Matrix(K*u) (u vector)
  H_sys_Middle : Gain  Gain=H_sys_Middle  Multiplication=Matrix(K*u) (u vector)
  H_sys_Middle1 : Gain  Gain=H_sys_Middle  Multiplication=Matrix(K*u) (u vector)
  Hd_Middle : Gain  Gain=Hd_Middle  Multiplication=Matrix(K*u) (u vector)
  Ld_Middle{,1..3} (4 alike) : Gain  Gain=Ld_Middle  Multiplication=Matrix(K*u) (u vector)
  Sum1 : Sum  Inputs=+-
  Sum2 : Sum  Inputs=+++
  Sum4 : Sum  Inputs=+++
  Sum5 : Sum  Inputs=+++
  Sum6 : Sum
  Sum7 : Sum  Inputs=-+
  velocity_sim : Outport
  yaw_sim : Outport  Port=2
  SystemError : Outport  Port=3
  Ldterm : Outport  Port=4
  OutputError : Outport  Port=5
  yhat : Outport  Port=6
  xh_simulator : Outport  Port=7
  wires:
  H_sys_Middle/1 -> Sum2/2
  D_out_Middle/1 -> Sum4/2
  Delay1/1 -> Gd_Middle/1
  u_simulator/1 -> Delay3/1, Delay2/1, H_sys_Middle1/1, H_sys_Middle/1
  Ld_Middle/1 -> Ldterm/1, Sum2/1
  G_sys_Middle1/1 -> Sum6/1
  Sum2/1 -> Delay/1
  C_Middle/1 -> Sum7/1
  H_sys_Middle1/1 -> Sum6/2
  Delay2/1 -> D_out_Middle/1
  Ref/1 -> Sum7/2
  Delay3/1 -> Hd_Middle/1
  Delay4/1 -> C_out_Middle/1
  Ld_Middle1/1 -> Sum5/1
  Delay/1 -> G_sys_Middle1/1, C_Middle1/1, G_sys_Middle/1, Delay4/1
  Hd_Middle/1 -> Sum5/2
  C_out_Middle/1 -> Sum4/3
  Sum5/1 -> xh_simulator/1, C_Middle2/1, Delay1/1
  Sum7/1 -> SystemError/1, Ld_Middle/1
  C_Middle1/1 -> Sum4/1
  G_sys_Middle/1 -> Sum2/3
  Sum6/1 -> C_Middle/1
  Gd_Middle/1 -> Sum5/3
  Demux/2 -> yaw_sim/1
  Demux/1 -> velocity_sim/1
  Sum4/1 -> Sum1/1, Demux/1, Ld_Middle1/1
  C_Middle2/1 -> yhat/1, Sum1/2
  Sum1/1 -> OutputError/1
  r(k-1)/1 -> Ld_Middle3/1
  Ld_Middle3/1 -> Delay4/2, Delay1/2
  r(k)/1 -> Ld_Middle2/1
  Ld_Middle2/1 -> Delay/2
  udelayFront/1 -> Delay2/2, Delay3/2

== system Copy_of_MPC_control/all_system/Middle_simulator1/VH2P ==
  Velocities : Inport
  HeadingAngles : Inport  Port=2
  PositionfromFront : Inport  Port=3
  VelocitiesfromFront : Inport  Port=4
  HeadingAnglesfromFront : Inport  Port=5
  T_sim : Inport  Port=6
  LastT_sim : Inport  Port=7
  Resettable Delay : Delay  DelayLength=1  InitialConditionSource=Input port  ExternalReset=Rising  SampleTime=Ts
      settings: InputPortMap=u0,r5,p4
  Resettable Delay1 : Delay  DelayLength=1  InitialConditionSource=Input port  ExternalReset=Rising  SampleTime=Ts
      settings: InputPortMap=u0,r5,p4
  Resettable Delay2 : Delay  DelayLength=1  InitialConditionSource=Input port  ExternalReset=Rising  SampleTime=Ts
      settings: InputPortMap=u0,r5,p4
  To Workspace : ToWorkspace  VariableName=positionfromfront  SampleTime=Ts
  To Workspace1 : ToWorkspace  VariableName=Hfromfront  SampleTime=Ts
  To Workspace2 : ToWorkspace  VariableName=Vfromfront  SampleTime=Ts
  Trigger : Subsystem
  YV2P : MATLAB Function  TreatAsAtomicUnit=on  SystemSampleTime=Ts
  Position : Outport
  wires:
  YV2P/1(Position) -> Resettable Delay/1, Position/1
  LastT_sim/1 -> YV2P/6(LastTsim)
  Velocities/1 -> YV2P/1(Velocity), Resettable Delay1/1
  Resettable Delay1/1 -> To Workspace2/1, YV2P/3(LastVelocity)
  HeadingAngles/1 -> YV2P/2(Yaw), Resettable Delay2/1
  Resettable Delay2/1 -> To Workspace1/1, YV2P/4(LastYaw)
  Resettable Delay/1 -> To Workspace/1, YV2P/7(Lastpostion)
  Trigger/1(Trig) -> Resettable Delay2/2, Resettable Delay1/2, Resettable Delay/2
  PositionfromFront/1 -> Resettable Delay/3
  HeadingAnglesfromFront/1 -> Resettable Delay2/3
  VelocitiesfromFront/1 -> Resettable Delay1/3
  T_sim/1 -> YV2P/5(Tsim)

== system Copy_of_MPC_control/all_system/Middle_simulator1/YV_update_Np ==
  XY_sim : Inport
  Velocity_sim : Inport  Port=2
  Heading_sim : Inport  Port=3
  From Workspace1 : FromWorkspace  VariableName=T_sim  SampleTime=Ts
  From Workspace3 : FromWorkspace  VariableName=XY_Ref_Upd  SampleTime=Ts
  MATLAB Function2 : MATLAB Function  TreatAsAtomicUnit=on  SystemSampleTime=Ts
  Unit Delay1 : UnitDelay  SampleTime=Ts
  Unit Delay4 : UnitDelay  SampleTime=Ts
  Unit Delay5 : UnitDelay  SampleTime=Ts
  Velocity : Outport
  Heading angle : Outport  Port=2
  wires:
  MATLAB Function2/1(Velocity_updated) -> Velocity/1
  From Workspace3/1 -> MATLAB Function2/1(XY_ref)
  MATLAB Function2/2(Heading_updated) -> Heading angle/1
  From Workspace1/1 -> MATLAB Function2/8(Tsim)
  XY_sim/1 -> Unit Delay1/1, MATLAB Function2/2(XY_sim)
  Velocity_sim/1 -> MATLAB Function2/4(Velocity_sim), Unit Delay5/1
  Heading_sim/1 -> MATLAB Function2/6(Yaw_sim), Unit Delay4/1
  Unit Delay1/1 -> MATLAB Function2/3(LastXY_sim)
  Unit Delay5/1 -> MATLAB Function2/5(LastVelocity_sim)
  Unit Delay4/1 -> MATLAB Function2/7(LastYaw_sim)

== system Copy_of_MPC_control/all_system/Mpc_block1/Extrapolation_select ==
  Clock14 : Clock
  Constant2 : Constant  Value=Timetochange2
  Constant3 : Constant  Value=Timetochange
  Select_model : MATLAB Function  TreatAsAtomicUnit=on  SystemSampleTime=Ts
  Select : Outport
  wires:
  Constant3/1 -> Select_model/2(Tc1)
  Constant2/1 -> Select_model/3(Tc2)
  Clock14/1 -> Select_model/1(Time)
  Select_model/1(Select) -> Select/1

== system Copy_of_MPC_control/all_system/Passenger Vehicle1/Body, Suspension, Wheels ==
  note: 1) Add Subsystem or Model blocks as valid variant choices.
      | 2) You cannot connect blocks at this level. At simulation, connectivity is automatically
      | determined, based on the active variant and port name matching.
  WindXYZ : Inport
  Ground : Inport  Port=2  PortDimensions=4
  Friction : Inport  Port=3  PortDimensions=4
  WheelAngle : Inport  Port=4
  AxleTrq : Inport  Port=5
  BrkPrs : Inport  Port=6
  PassVeh14DOF : ModelReference  DisableCoverage=on  ModelNameDialog=PassVeh14DOF  VariantControl=3  ModelReferenceVersion=1.200
  PassVeh7DOF : ModelReference  DisableCoverage=on  ModelNameDialog=PassVeh7DOF  VariantControl=1  ModelReferenceVersion=1.152
  xdot : Outport
  ydot : Outport  Port=2
  X : Outport  Port=3
  Y : Outport  Port=4
  Z : Outport  Port=5
  Xdot : Outport  Port=6
  Ydot : Outport  Port=7
  phi : Outport  Port=8
  theta : Outport  Port=9
  psi : Outport  Port=10
  p : Outport  Port=11
  q : Outport  Port=12
  r : Outport  Port=13
  ay : Outport  Port=14
  kappa : Outport  Port=15
  zAxle : Outport  Port=16
  omega : Outport  Port=17
  ZHP : Outport  Port=18  Unit=m
  XWheel : Outport  Port=19
  YWheel : Outport  Port=20

== system Copy_of_MPC_control/all_system/Passenger Vehicle1/Engine ==
  note: 1) Add Subsystem or Model blocks as valid variant choices.
      | 2) You cannot connect blocks at this level. At simulation, connectivity is automatically
      | determined, based on the active variant and port name matching.
  TrqCmd : Inport
  EngSpd : Inport  Port=2  Unit=rad/s
  Ideal Mapped Engine : ModelReference  DisableCoverage=on  ModelNameDialog=SiMappedEngineV  VariantControl=0  ModelReferenceVersion=1.335
  EngTrq : Outport

== system Copy_of_MPC_control/all_system/Passenger Vehicle1/Steering, Transmission, Driveline and Brakes ==
  note: 1) Add Subsystem or Model blocks as valid variant choices.
      | 2) You cannot connect blocks at this level. At simulation, connectivity is automatically
      | determined, based on the active variant and port name matching.
  SteerHWCmd : Inport
  EngTrq : Inport  Port=2
  GearCmd : Inport  Port=3  OutDataTypeStr=int8
  BrkPrsCmd : Inport  Port=4  PortDimensions=4
  omega : Inport  Port=5
  Driveline Ideal Fixed Gear : ModelReference  DisableCoverage=on  ModelNameDialog=Driveline  VariantControl=0  ModelReferenceVersion=1.207
  WhlAng : Outport
  AxlTrq : Outport  Port=2
  BrkPrs : Outport  Port=3  PortDimensions=4
  EngSpd : Outport  Port=4  Unit=rad/s
  PropShftSpd : Outport  Port=5

== system Copy_of_MPC_control/all_system/Passenger Vehicle1/Subsystem ==
  Env : Inport
  Driveline : Inport  Port=2
  Bus Selector1 : BusSelector  OutputSignals=Gnd.z.G_FL_z,Gnd.z.G_FR_z,Gnd.z.G_RL_z,Gnd.z.G_RR_z
  Bus Selector2 : BusSelector  OutputSignals=Wind
  Bus Selector3 : BusSelector  OutputSignals=Gnd.mu.mu_FL,Gnd.mu.mu_FR,Gnd.mu.mu_RL,Gnd.mu.mu_RR
  Bus Selector4 : BusSelector  OutputSignals=WhlAng,AxlTrq,BrkPrs
  Vector Concatenate : Concatenate  NumInputs=4
  Vector Concatenate1 : Concatenate  NumInputs=4
  Wind : Outport
  Gnd : Outport  Port=2
  mu : Outport  Port=3
  WhlAng : Outport  Port=4
  AxleTrq : Outport  Port=5
  BrkPrs : Outport  Port=6
  wires:
  Env/1 -> Bus Selector3/1, Bus Selector1/1, Bus Selector2/1
  Bus Selector2/1 -> Wind/1  "<Wind>"
  Bus Selector3/1 -> Vector Concatenate/1  "<mu_FL>"
  Bus Selector3/2 -> Vector Concatenate/2  "<mu_FR>"
  Bus Selector3/3 -> Vector Concatenate/3  "<mu_RL>"
  Bus Selector3/4 -> Vector Concatenate/4  "<mu_RR>"
  Vector Concatenate/1 -> mu/1
  Bus Selector1/1 -> Vector Concatenate1/1  "<G_FL_z>"
  Bus Selector1/2 -> Vector Concatenate1/2  "<G_FR_z>"
  Bus Selector1/3 -> Vector Concatenate1/3  "<G_RL_z>"
  Bus Selector1/4 -> Vector Concatenate1/4  "<G_RR_z>"
  Vector Concatenate1/1 -> Gnd/1
  Driveline/1 -> Bus Selector4/1
  Bus Selector4/2 -> AxleTrq/1  "<AxlTrq>"
  Bus Selector4/1 -> WhlAng/1  "<WhlAng>"
  Bus Selector4/3 -> BrkPrs/1  "<BrkPrs>"

== system Copy_of_MPC_control/all_system/Passenger Vehicle1/Subsystem1 ==
  WhlAng : Inport
  AxlTrq : Inport  Port=2
  BrkPrs : Inport  Port=3
  EngSpd : Inport  Port=4
  PropShftSpd : Inport  Port=5
  Bus Creator1 : BusCreator  Inputs=5
  Driveline : Outport
  wires:
  Bus Creator1/1 -> Driveline/1  "Driveline"
  PropShftSpd/1 -> Bus Creator1/5  "PropShftSpd"
  AxlTrq/1 -> Bus Creator1/2  "AxlTrq"
  WhlAng/1 -> Bus Creator1/1  "WhlAng"
  EngSpd/1 -> Bus Creator1/4  "EngSpd"
  BrkPrs/1 -> Bus Creator1/3  "BrkPrs"

== system Copy_of_MPC_control/all_system/Passenger Vehicle1/Subsystem2 ==
  Cntrl : Inport
  SteerCmd : Inport  Port=2
  EngTrqCmd : Inport  Port=3
  Wheels : Inport  Port=4
  Bus Selector1 : BusSelector  OutputSignals=Steer
  Bus Selector2 : BusSelector  OutputSignals=omega
  Bus Selector3 : BusSelector  OutputSignals=Transmission.GearCmd,Brake.PrsCmd
  Bus Selector4 : BusSelector  OutputSignals=EngTrq
  Steer : Outport
  EngTrq : Outport  Port=2
  GearCmd : Outport  Port=3
  PrsCmd : Outport  Port=4
  omega : Outport  Port=5
  wires:
  Cntrl/1 -> Bus Selector3/1
  Bus Selector3/1 -> GearCmd/1  "<GearCmd>"
  SteerCmd/1 -> Bus Selector1/1
  Wheels/1 -> Bus Selector2/1
  Bus Selector2/1 -> omega/1  "<omega>"
  Bus Selector3/2 -> PrsCmd/1  "<PrsCmd>"
  EngTrqCmd/1 -> Bus Selector4/1
  Bus Selector1/1 -> Steer/1  "<Steer>"
  Bus Selector4/1 -> EngTrq/1  "<EngTrq>"

== system Copy_of_MPC_control/all_system/Passenger Vehicle1/Subsystem3 ==
  Cntrl : Inport
  Driveline : Inport  Port=2
  Bus Selector : BusSelector  OutputSignals=ECU.EngTrqCmd
  Bus Selector1 : BusSelector  OutputSignals=EngSpd
  EngTrqCmd : Outport
  EngSpd : Outport  Port=2
  wires:
  Driveline/1 -> Bus Selector1/1
  Cntrl/1 -> Bus Selector/1
  Bus Selector/1 -> EngTrqCmd/1  "<EngTrqCmd>"
  Bus Selector1/1 -> EngSpd/1  "<EngSpd>"

== system Copy_of_MPC_control/all_system/Passenger Vehicle1/Subsystem4 ==
  xdot : Inport
  ydot : Inport  Port=2
  X : Inport  Port=3
  Y : Inport  Port=4
  Z : Inport  Port=5
  Xdot : Inport  Port=6
  Ydot : Inport  Port=7
  phi : Inport  Port=8
  theta : Inport  Port=9
  psi : Inport  Port=10
  p : Inport  Port=11
  q : Inport  Port=12
  r : Inport  Port=13
  ay : Inport  Port=14
  kappa : Inport  Port=15
  zAxle : Inport  Port=16
  omega : Inport  Port=17
  ZHP : Inport  Port=18
  XWheel : Inport  Port=19
  YWheel : Inport  Port=20
  Bus Creator : BusCreator  Inputs=15
  Bus Creator3 : BusCreator  Inputs=5
  Chassis : Outport
  Wheels : Outport  Port=2
  wires:
  X/1 -> Bus Creator/3  "X"
  psi/1 -> Bus Creator/10  "psi"
  ydot/1 -> Bus Creator/2  "ydot"
  Z/1 -> Bus Creator/5  "Z"
  Bus Creator/1 -> Chassis/1  "Chassis"
  Y/1 -> Bus Creator/4  "Y"
  xdot/1 -> Bus Creator/1  "xdot"
  r/1 -> Bus Creator/13  "r"
  ay/1 -> Bus Creator/14  "ay"
  omega/1 -> Bus Creator3/3  "omega"
  zAxle/1 -> Bus Creator3/2  "zAxle"
  kappa/1 -> Bus Creator3/1  "kappa"
  Bus Creator3/1 -> Wheels/1  "Wheels"
  theta/1 -> Bus Creator/9  "theta"
  phi/1 -> Bus Creator/8  "phi"
  Xdot/1 -> Bus Creator/6  "Xdot"
  Ydot/1 -> Bus Creator/7  "Ydot"
  ZHP/1 -> Bus Creator/15  "ZHP"
  p/1 -> Bus Creator/11  "p"
  q/1 -> Bus Creator/12  "q"
  YWheel/1 -> Bus Creator3/5  "YWheel"
  XWheel/1 -> Bus Creator3/4  "XWheel"

== system Copy_of_MPC_control/all_system/Passenger Vehicle1/Subsystem5 ==
  "EngTrq " : Inport
  Bus Creator : BusCreator  Inputs=1
  Eng : Outport
  wires:
  "EngTrq "/1 -> Bus Creator/1  "EngTrq"
  Bus Creator/1 -> Eng/1

== system Copy_of_MPC_control/all_system/Subsystem2/Dataselect ==
  Clock15 : Clock
  Constant3 : Constant  Value=Statechange
  Constant4 : Constant  Value=Statechange2
  Dataselect : MATLAB Function  TreatAsAtomicUnit=on
  DS : Outport
  wires:
  Constant4/1 -> Dataselect/3(Statechange2)
  Clock15/1 -> Dataselect/1(timing)
  Constant3/1 -> Dataselect/2(Statechange)
  Dataselect/1(select) -> DS/1

== system Copy_of_MPC_control/all_system/Visualization1/3D Engine ==
  note: 1) Add Subsystem or Model blocks as valid variant choices.
      | 2) You cannot connect blocks at this level. At simulation, connectivity is automatically
      | determined, based on the active variant and port name matching.
  VehFdbk : Inport
  3D Engine : Subsystem  VariantControl=1
  3D Engine Disabled : Subsystem  VariantControl=0

== system Copy_of_MPC_control/all_system/Visualization1/Acceleration Cmd ==

== system Copy_of_MPC_control/all_system/Visualization1/Brake Cmd ==

== system Copy_of_MPC_control/all_system/Visualization1/Engine Tach [rpm] ==

== system Copy_of_MPC_control/all_system/Visualization1/Handwheel Angle [deg] ==

== system Copy_of_MPC_control/all_system/Visualization1/Lateral Acceleration [g] ==

== system Copy_of_MPC_control/all_system/Visualization1/Speed [mph] ==

== system Copy_of_MPC_control/all_system/Visualization1/Vehicle XY Plotter ==
  VehFdbk : Inport
  Bus Selector1 : BusSelector  OutputSignals=Body.phi,Body.theta,Body.psi  OutputAsBus=on
  Bus Selector2 : BusSelector  OutputSignals=Driveline.WhlAng  OutputAsBus=on
  Bus Selector3 : BusSelector  OutputSignals=Body.X,Body.Y,Body.Z  OutputAsBus=on
  Bus Selector4 : BusSelector  OutputSignals=Body.Xdot,Body.Ydot  OutputAsBus=on
  Bus to Vector{,1..3} (4 alike) : BusToVector
  Ground : Ground
  Rate Transition{1..2,5..6} (4 alike) : RateTransition  OutPortSampleTime=pltDT
  Vector Concatenate : Concatenate
  Vehicle XY Plotter : vehdynlibviscommon/Vehicle XY Plotter  bufferSize=bufferSize  w=w  a=a  b=b
  wires:
  Bus to Vector2/1 -> Rate Transition1/1  "InertCGDisp"
  Rate Transition5/1 -> Vehicle XY Plotter/1
  Bus Selector4/1 -> Bus to Vector1/1
  Rate Transition1/1 -> Vehicle XY Plotter/2
  Rate Transition6/1 -> Vehicle XY Plotter/3
  Vector Concatenate/1 -> Rate Transition6/1  "InertCGVel"
  Bus Selector1/1 -> Bus to Vector2/1
  Bus to Vector/1 -> Rate Transition5/1  "InertCGDisp"
  Bus Selector3/1 -> Bus to Vector/1
  Bus to Vector1/1 -> Vector Concatenate/1
  Ground/1 -> Vector Concatenate/2
  Bus to Vector3/1 -> Rate Transition2/1
  Bus Selector2/1 -> Bus to Vector3/1
  VehFdbk/1 -> Bus Selector1/1, Bus Selector2/1, Bus Selector4/1, Bus Selector3/1
  Rate Transition2/1 -> Vehicle XY Plotter/4

== system Copy_of_MPC_control/observer/simulator_1/Mpc_Simulator_Middle ==
  Velocity_updated : Inport  SampleTime=Ts  LockScale=on
  Heading_updated : Inport  Port=2  SampleTime=Ts  LockScale=on
  Xhat : Inport  Port=3
  Clock : Clock
  Constant1 : Constant  Value=M  VectorParams1D=off  SampleTime=-1
  Constant2 : Constant  Value=Np  SampleTime=-1
  Constant4 : Constant  Value=Qc  VectorParams1D=off  SampleTime=-1
  Constant5 : Constant  Value=phi_Front_1  VectorParams1D=off  SampleTime=-1
  Constant6 : Constant  Value=JE_Front_1  VectorParams1D=off  SampleTime=-1
  F_Middle : Gain  Gain=F_Front_1  Multiplication=Matrix(K*u) (u vector)
  From Workspace1 : FromWorkspace  VariableName=select_MPC  SampleTime=Ts
  From Workspace6 : FromWorkspace  VariableName=Rs  SampleTime=Ts
  MATLAB Function : MATLAB Function  TreatAsAtomicUnit=on  SystemSampleTime=Ts
  Unit Delay : UnitDelay  InitialCondition=[0;0]  SampleTime=Ts
  U : Outport
  r : Outport  Port=2
  wires:
  Unit Delay/1 -> MATLAB Function/12(U_delay)
  MATLAB Function/2(U) -> Unit Delay/1, U/1
  Xhat/1 -> F_Middle/1
  Constant4/1 -> MATLAB Function/4(Qc)
  Constant5/1 -> MATLAB Function/2(phi)
  Constant6/1 -> MATLAB Function/1(JE)
  Constant2/1 -> MATLAB Function/6(Np)
  Constant1/1 -> MATLAB Function/5(M)
  Clock/1 -> MATLAB Function/10(Tsim)
  F_Middle/1 -> MATLAB Function/3(Fxh)
  From Workspace6/1 -> MATLAB Function/9(Rs)
  Heading_updated/1 -> MATLAB Function/7(Heading_updated)
  Velocity_updated/1 -> MATLAB Function/8(Velocity_updated)
  MATLAB Function/1(r) -> r/1
  From Workspace1/1 -> MATLAB Function/11(select_MPC)
